simulink model "ModelOfCraneComponentDiscrete"  (R2017b)
settings: Solver=FixedStepDiscrete  StartTime=0.0  StopTime=10.0  FixedStep=0.01  RelTol=1e-3
values from neighbouring files (symbols this model uses):
  discretePendulumModel = c2d(continuousPendulumModel, 1/100)    [GlobalVariables.m]
  discreteSledgeModel = c2d(continuousSledgeModel, 1/100)    [GlobalVariables.m]
  Dp = 0.007    [GlobalVariables.m]    (also in GlobalVariables.mat = 0.0013905996261; Workspace_stuff.m)
  Dsm = 62.892    [GlobalVariables.m]    (also in GlobalVariables.mat = 4.80816522254)
  g = 9.82    [GlobalVariables.m]    (also in GlobalVariables.mat; Workspace_stuff.m)
  Jp = 0.016    [GlobalVariables.m]    (also in GlobalVariables.mat = 0.0135518532857; Workspace_stuff.m = 0.0130478452133)
  ke = 0.1377    [GlobalVariables.m]    (also in GlobalVariables.mat = 0.00328754355818)
  kt = 0.138    [GlobalVariables.m]    (also in GlobalVariables.mat = 0.0136303622306)
  Lcm = Lr + hl/2    (= 0.2485)    [GlobalVariables.m]    (also in GlobalVariables.mat; Workspace_stuff.m)
  Lr = 24.1/100    (= 0.241)    [GlobalVariables.m]    (also in GlobalVariables.mat; Workspace_stuff.m)
  mj = ms * Jm    (= 2.0274e-05)    [GlobalVariables.m]    (also in GlobalVariables.mat = 7.2062003e-08)
  ml = 0.184    [GlobalVariables.m]    (also in GlobalVariables.mat; Workspace_stuff.m)
  mr = 0.085    [GlobalVariables.m]    (also in GlobalVariables.mat; Workspace_stuff.m)
  Ra = 4.2    [GlobalVariables.m]    (also in GlobalVariables.mat; Workspace_stuff.m)
  rm = 0.7/100    (= 0.007)    [GlobalVariables.m]    (also in GlobalVariables.mat; Workspace_stuff.m)
settings Model: Creator=labadmin  LastModifiedBy=labadmin
settings DataIOCC: SaveOutput=off  SaveTime=off

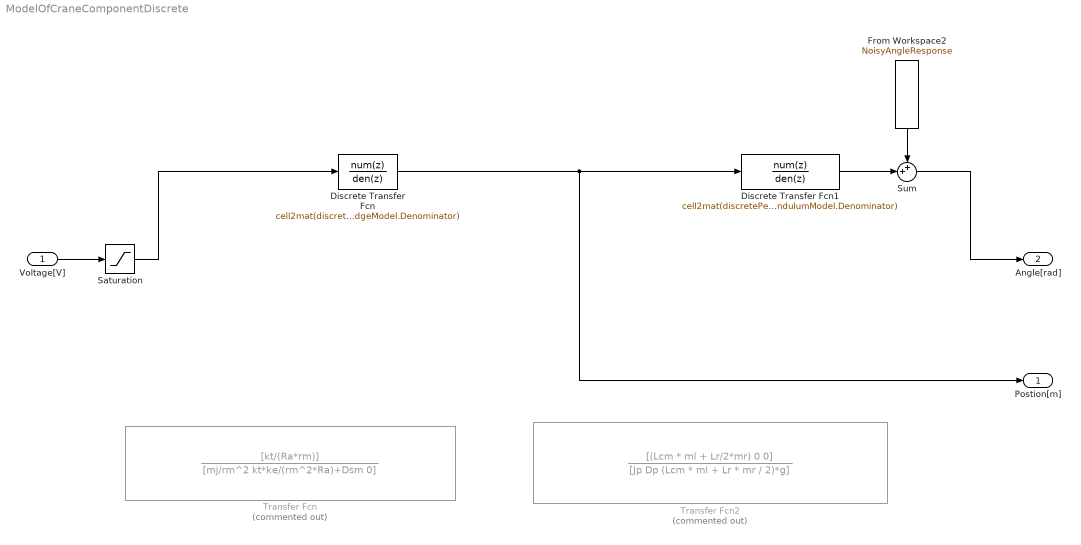
== system ModelOfCraneComponentDiscrete ==
  Voltage[V] : Inport  OutDataTypeStr=double  PortDimensions=1
  Discrete Transfer Fcn : DiscreteTransferFcn  Numerator=cell2mat(discreteSledgeModel.Numerator)  Denominator=cell2mat(discreteSledgeModel.Denominator)
  Discrete Transfer Fcn1 : DiscreteTransferFcn  Numerator=cell2mat(discretePendulumModel.Numerator)  Denominator=cell2mat(discretePendulumModel.Denominator)
  From Workspace2 : FromWorkspace  VariableName=NoisyAngleResponse
  Saturation : Saturate  UpperLimit=6-1.4  LowerLimit=-6+1.4
  Sum : Sum  Inputs=++|
  Transfer Fcn : TransferFcn  Commented=on  Numerator=[kt/(Ra*rm)]  Denominator=[mj/rm^2 kt*ke/(rm^2*Ra)+Dsm 0]
  Transfer Fcn2 : TransferFcn  Commented=on  Numerator=[(Lcm * ml + Lr/2*mr) 0 0]  Denominator=[Jp Dp (Lcm * ml + Lr * mr / 2)*g]
  "Postion[m] " : Outport  SignalName=Position[m]  OutDataTypeStr=double  PortDimensions=1  SampleTime=0
  Angle[rad] : Outport  Port=2  SignalName=Angle[rad]  OutDataTypeStr=double  PortDimensions=1  SampleTime=0
  wires:
  Saturation/1 -> Discrete Transfer Fcn/1
  Voltage[V]/1 -> Saturation/1
  Discrete Transfer Fcn/1 -> "Postion[m] "/1, Discrete Transfer Fcn1/1
  Discrete Transfer Fcn1/1 -> Sum/2
  From Workspace2/1 -> Sum/1
  Sum/1 -> Angle[rad]/1
